simulink subsystem "battery_charger"  (R2021a)
settings: Solver=VariableStepAuto  StartTime=0.0  StopTime=10.0  RelTol=1e-3
libraries: fl_lib x4, nesl_utility x2, ee_lib x1
settings Model: Creator=Carlo Edoardo  LastModifiedBy=Carlo Edoardo

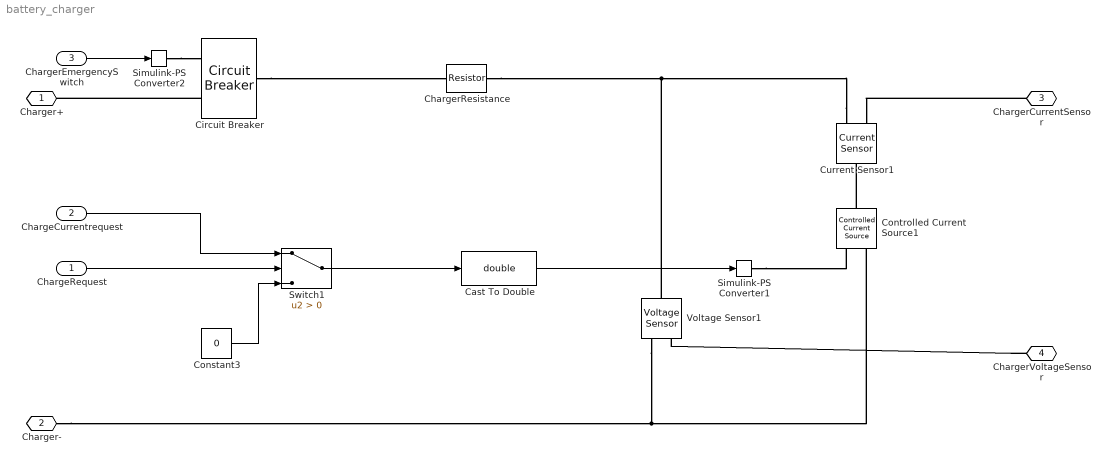
== system battery_charger ==
  ChargeRequest : Inport
  ChargeCurrentrequest : Inport  Port=2
  ChargerEmergencySwitch : Inport  Port=3
  Cast To Double : DataTypeConversion  OutDataTypeStr=double
  ChargerResistance : fl_lib/Electrical/Electrical Elements/Resistor  R=0 Ohm  i_specify=off  i_priority=None  i=0 A  i_nominal_specify=off  i_nominal_unit=A  i_nominal_value=1  v_specify=off  v_priority=None  v=0 V  v_nominal_specify=off  v_nominal_unit=V  v_nominal_value=1
  Circuit Breaker : ee_lib/Switches & Breakers/Circuit Breaker  R_closed=0.001 Ohm  G_open=1e-6 1/Ohm  threshold=0.5 V  offset_for_on=1 V
      settings: SourceProductBaseCode=PS  InternalSimscapePortConfiguration="{\"Bottom\":[],\"Left\":[{\"id\":\"vT\",\"label\":\"vT\",\"type\":\"input\"},{\"id\":\"p1\",\"label\":\"\",\"type\":\"foundation.electrical.electrical\"}],\"Right\":[{\"id\":\"p2\",\"label\":\"\",\"type\":\"foundation.electrical.electrical\"}],\"Top\":[]}"
  Constant3 : Constant  Value=0
  Controlled Current Source1 : fl_lib/Electrical/Electrical Sources/Controlled Current Source
  Current Sensor1 : fl_lib/Electrical/Electrical Sensors/Current Sensor
  Simulink-PS Converter1 : nesl_utility/Simulink-PS Converter  PhysicalDomain=network_engine_domain  SubClassName=ps_input  LeftPortType=input  RightPortType=output  PseudoPeriodic=off  Frequencies=[]  NoiseDistribution=none  NoiseParameters=[]  Unit=1  AffineConversion=off  FilteringAndDerivatives=provide  SimscapeFilterOrder=1  InputFilterTimeConstant=0.001  UdotUserProvided=0
      settings: SourceProductBaseCode=PW,SS
  Simulink-PS Converter2 : nesl_utility/Simulink-PS Converter  PhysicalDomain=network_engine_domain  SubClassName=ps_input  LeftPortType=input  RightPortType=output  PseudoPeriodic=off  Frequencies=[]  NoiseDistribution=none  NoiseParameters=[]  Unit=1  AffineConversion=off  FilteringAndDerivatives=provide  SimscapeFilterOrder=1  InputFilterTimeConstant=0.001  UdotUserProvided=0
      settings: SourceProductBaseCode=PW,SS
  Switch1 : Switch  Criteria=u2 > Threshold
  Voltage Sensor1 : fl_lib/Electrical/Electrical Sensors/Voltage Sensor
  Charger+ : PMIOPort  Side=Left
  Charger- : PMIOPort  Port=2  Side=Left
  ChargerCurrentSensor : PMIOPort  Port=3  Side=Right
  ChargerVoltageSensor : PMIOPort  Port=4  Side=Right
  wires:
  ChargeRequest/1 -> Switch1/2
  ChargerEmergencySwitch/1 -> Simulink-PS Converter2/1
  Constant3/1 -> Switch1/3
  Switch1/1 -> Cast To Double/1
  Cast To Double/1 -> Simulink-PS Converter1/1
  ChargeCurrentrequest/1 -> Switch1/1
  connections:
  Current Sensor1/RConn2 -- Voltage Sensor1/LConn1 -- ChargerResistance/RConn1
  Voltage Sensor1/RConn2 -- Charger-/RConn1 -- Controlled Current Source1/RConn2
  ChargerVoltageSensor/RConn1 -- Voltage Sensor1/RConn1
  Simulink-PS Converter1/RConn1 -- Controlled Current Source1/RConn1
  Controlled Current Source1/LConn1 -- Current Sensor1/LConn1
  Circuit Breaker/RConn1 -- ChargerResistance/LConn1
  Simulink-PS Converter2/RConn1 -- Circuit Breaker/LConn1
  Circuit Breaker/LConn2 -- Charger+/RConn1
  ChargerCurrentSensor/RConn1 -- Current Sensor1/RConn1
